simulink model "AMKSpeedLimit"  (R2019b)
settings: Solver=VariableStepAuto  StartTime=0.0  StopTime=10.0  RelTol=1e-3
libraries: simulink x4
settings Model: Creator=12045  LastModifiedBy=12045

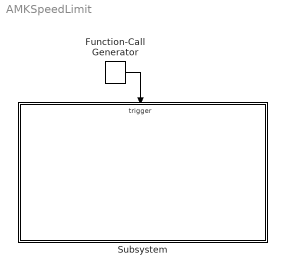
== system AMKSpeedLimit ==
  Function-Call Generator : simulink/Ports & Subsystems/Function-Call Generator  sample_time=0.01  numberOfIterations=1
  Subsystem : Subsystem
  wires:
  Function-Call Generator/1 -> Subsystem/Trigger

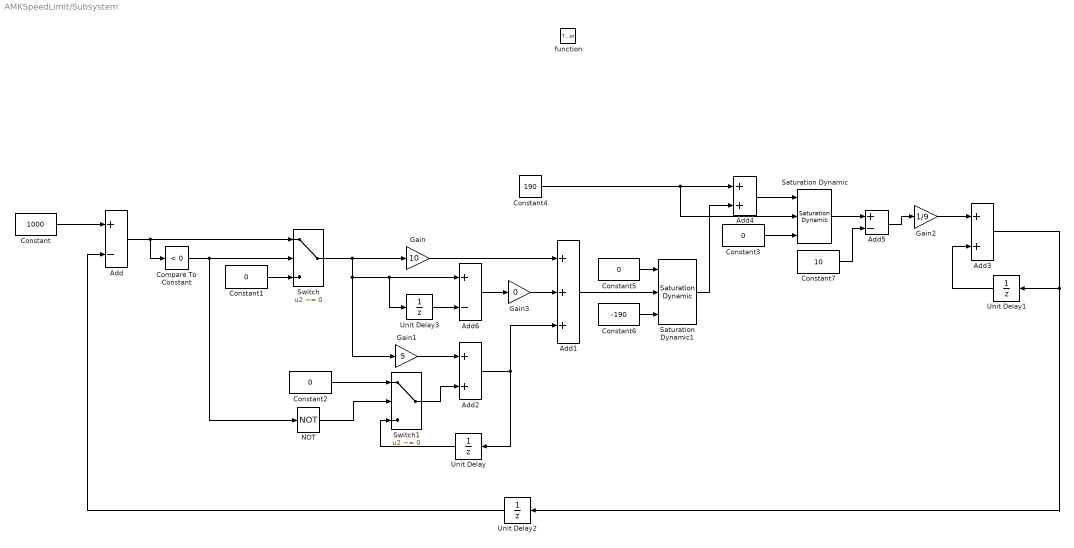
== system AMKSpeedLimit/Subsystem ==
  function : TriggerPort  TriggerType=function-call  VariantControl=Variant
  Add : Sum  Inputs=+-
  Add1 : Sum  Inputs=+++
  Add2 : Sum
  Add3 : Sum
  Add4 : Sum
  Add5 : Sum  Inputs=+-
  Add6 : Sum  Inputs=+-
  Compare To Constant : simulink/Logic and Bit Operations/Compare To Constant  relop=<  const=0  OutDataTypeStr=boolean
  Constant : Constant  Value=1000
  Constant{1..3,5} (4 alike) : Constant  Value=0
  Constant4 : Constant  Value=190
  Constant6 : Constant  Value=-190
  Constant7 : Constant  Value=10
  Gain : Gain  Gain=10
  Gain1 : Gain  Gain=5
  Gain2 : Gain  Gain=1/9
  Gain3 : Gain  Gain=0
  NOT : Logic  Operator=NOT  AllPortsSameDT=off  OutDataTypeStr=boolean
  Saturation Dynamic : simulink/Discontinuities/Saturation Dynamic  OutMin=[]  OutMax=[]  OutDataTypeStr=Inherit: Same as second input  OutDataType=fixdt(1, 16)  OutScaling=2^-10  DoSatur=off
  Saturation Dynamic1 : simulink/Discontinuities/Saturation Dynamic  OutMin=[]  OutMax=[]  OutDataTypeStr=Inherit: Same as second input  OutDataType=fixdt(1, 16)  OutScaling=2^-10  DoSatur=off
  Switch : Switch  Criteria=u2 ~= 0
  Switch1 : Switch  Criteria=u2 ~= 0
  Unit Delay{,1..3} (4 alike) : UnitDelay  SampleTime=-1  HasFrameUpgradeWarning=on
  wires:
  Constant/1 -> Add/1
  Add/1 -> Switch/1, Compare To Constant/1
  Compare To Constant/1 -> NOT/1, Switch/2
  Constant1/1 -> Switch/3
  Switch/1 -> Gain1/1, Unit Delay3/1, Add6/1, Gain/1
  Gain/1 -> Add1/1
  Gain1/1 -> Add2/1
  Add2/1 -> Unit Delay/1, Add1/3
  Unit Delay/1 -> Switch1/3
  Switch1/1 -> Add2/2
  NOT/1 -> Switch1/2
  Constant2/1 -> Switch1/1
  Constant4/1 -> Saturation Dynamic/2, Add4/1
  Add3/1 -> Unit Delay1/1, Unit Delay2/1
  Unit Delay1/1 -> Add3/2
  Gain2/1 -> Add3/1
  Saturation Dynamic/1 -> Add5/1
  Add1/1 -> Saturation Dynamic1/2
  Unit Delay2/1 -> Add/2
  Saturation Dynamic1/1 -> Add4/2
  Unit Delay3/1 -> Add6/2
  Add6/1 -> Gain3/1
  Gain3/1 -> Add1/2
  Add4/1 -> Saturation Dynamic/1
  Constant3/1 -> Saturation Dynamic/3
  Constant5/1 -> Saturation Dynamic1/1
  Constant6/1 -> Saturation Dynamic1/3
  Constant7/1 -> Add5/2
  Add5/1 -> Gain2/1
